simulink model "Reg_Obs2"  (R2017b)
settings: Solver=VariableStepAuto  StartTime=0.0  StopTime=15  RelTol=1e-3
values from neighbouring files (symbols this model uses):
  kd = Q'\(a-az)    [Regul_Luenbergh2.m]    (also in Regul_Modal2.m)
  L1 = -((T'*Sn')^(-1))*(az-az_nab)    [Regul_Luenbergh2.m]
undefined symbols (not defined in the file or in its folder): Ad, Bd, Cd, Dd
settings Model: Creator=ASUS_302  LastModifiedBy=ASUS_302

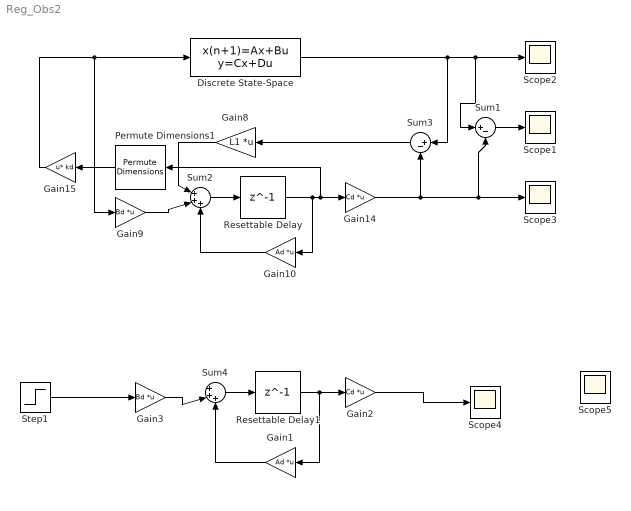
== system Reg_Obs2 ==
  Discrete State-Space : DiscreteStateSpace  A=Ad  B=Bd  C=Cd  D=Dd  InitialCondition=[1;1;1;1;0]  SampleTime=0.1
  Gain1 : Gain  Gain=Ad  Multiplication=Matrix(K*u)
  Gain10 : Gain  Gain=Ad  Multiplication=Matrix(K*u)
  Gain14 : Gain  Gain=Cd  Multiplication=Matrix(K*u)
  Gain15 : Gain  Gain=kd  Multiplication=Matrix(u*K)
  Gain2 : Gain  Gain=Cd  Multiplication=Matrix(K*u)
  Gain3 : Gain  Gain=Bd  Multiplication=Matrix(K*u)
  Gain8 : Gain  Gain=L1  Multiplication=Matrix(K*u)
  Gain9 : Gain  Gain=Bd  Multiplication=Matrix(K*u)
  Permute Dimensions1 : PermuteDimensions
  Resettable Delay : Delay  DelayLength=1  InitialCondition=[1;1;1;1;1]  SampleTime=0.1
  Resettable Delay1 : Delay  DelayLength=1  InitialCondition=[1;1;1;1;1]
  Scope{1..5} (5 alike) : Scope
  Step1 : Step  Time=0.01  SampleTime=0
  Sum1 : Sum  Inputs=|+-
  Sum2 : Sum  Inputs=|+++
  Sum3 : Sum  Inputs=|+-
  Sum4 : Sum  Inputs=|+++
  wires:
  Permute Dimensions1/1 -> Gain15/1
  Sum3/1 -> Gain8/1
  Gain10/1 -> Sum2/3
  Gain9/1 -> Sum2/2
  Gain14/1 -> Sum1/2, Scope3/1, Sum3/2
  Discrete State-Space/1 -> Sum3/1, Sum1/1, Scope2/1
  Sum2/1 -> Resettable Delay/1
  Resettable Delay/1 -> Gain10/1, Permute Dimensions1/1, Gain14/1
  Resettable Delay1/1 -> Gain1/1, Gain2/1
  Sum4/1 -> Resettable Delay1/1
  Gain3/1 -> Sum4/2
  Gain1/1 -> Sum4/3
  Gain2/1 -> Scope4/1
  Step1/1 -> Gain3/1
  Gain15/1 -> Gain9/1, Discrete State-Space/1
  Gain8/1 -> Sum2/1
  Sum1/1 -> Scope1/1
